simulink subsystem "MPC3_nlpsol_ipopt"  (R2023b)
settings: Solver=VariableStepAuto  StartTime=0.0  StopTime=10.0  RelTol=1e-3
undefined symbols (not defined in the file): param_MPC3_ipopt_nlpsol, param_weight_MPC3_ipopt_nlpsol, parMHE
settings Model: Creator=emu  LastModifiedBy=emu

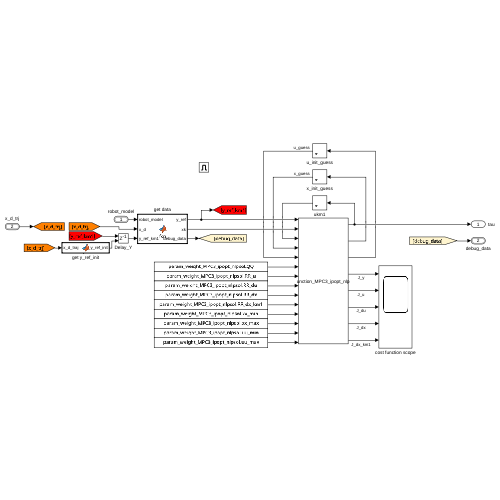
[thumbnail: Simulink's stored preview of the top-level diagram]
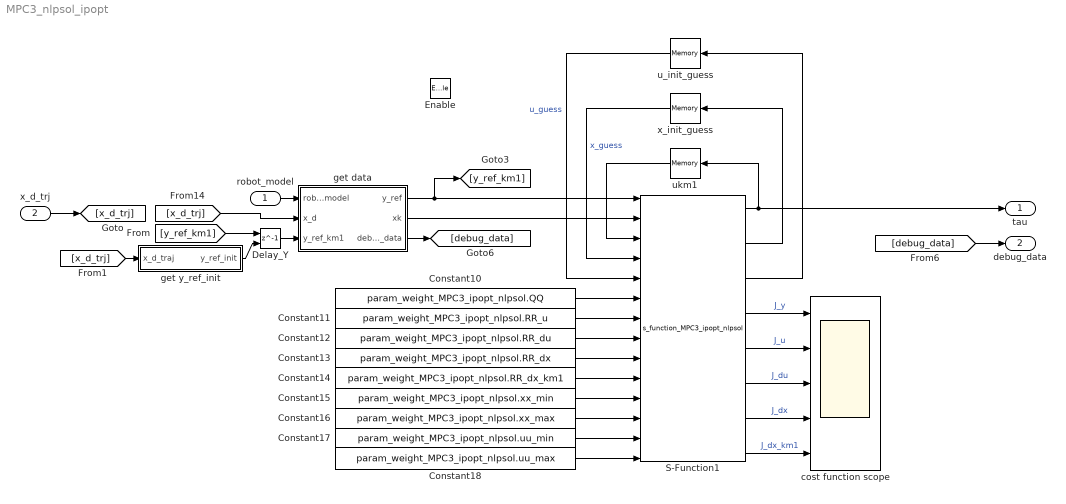
== system MPC3_nlpsol_ipopt ==
  robot_model : Inport  OutDataTypeStr=Bus: robot_model
  x_d_trj : Inport  Port=2  OutDataTypeStr=Bus: x_d
  Enable : EnablePort
  Constant10 : Constant  Value=param_weight_MPC3_ipopt_nlpsol.QQ
  Constant11 : Constant  Value=param_weight_MPC3_ipopt_nlpsol.RR_u
  Constant12 : Constant  Value=param_weight_MPC3_ipopt_nlpsol.RR_du
  Constant13 : Constant  Value=param_weight_MPC3_ipopt_nlpsol.RR_dx
  Constant14 : Constant  Value=param_weight_MPC3_ipopt_nlpsol.RR_dx_km1
  Constant15 : Constant  Value=param_weight_MPC3_ipopt_nlpsol.xx_min
  Constant16 : Constant  Value=param_weight_MPC3_ipopt_nlpsol.xx_max
  Constant17 : Constant  Value=param_weight_MPC3_ipopt_nlpsol.uu_min
  Constant18 : Constant  Value=param_weight_MPC3_ipopt_nlpsol.uu_max
  Delay_Y : Delay  DelayLength=1  InitialConditionSource=Input port  InitialCondition=zeros(parMHE.N*parMHE.n_y,1)
      settings: InputPortMap=u0,p4
  S-Function1 : S-Function  FunctionName=s_function_MPC3_ipopt_nlpsol  Parameters='s_functions/MPC3_ipopt_nlpsol.casadi', 'MPC3_ipopt_nlpsol'  SFunctionDeploymentMode=off  EnableBusSupport=off
  cost function scope : Scope  NumInputPorts=5
  get data : MATLAB Function  TreatAsAtomicUnit=on
  get y_ref_init : MATLAB Function  TreatAsAtomicUnit=on
  u_init_guess : Memory  InitialCondition=param_MPC3_ipopt_nlpsol.u_init_guess
  ukm1 : Memory  InitialCondition=param_MPC3_ipopt_nlpsol.u_init_guess(:,1)
  x_init_guess : Memory  InitialCondition=param_MPC3_ipopt_nlpsol.x_init_guess
  tau : Outport
  debug_data : Outport  Port=2  OutDataTypeStr=Bus: debug_data_bus
  wires:
  Constant15/1 -> S-Function1/11
  [y_ref_km1] -> Delay_Y/1
  u_init_guess/1 -> S-Function1/5  "u_guess"
  [x_d_trj] -> get y_ref_init/1(x_d_traj)
  Constant11/1 -> S-Function1/7
  S-Function1/1 -> ukm1/1, tau/1
  get data/1(y_ref) -> S-Function1/1, [y_ref_km1]
  x_d_trj/1 -> [x_d_trj]
  robot_model/1 -> get data/1(robot_model)
  get data/3(debug_data) -> [debug_data]
  [debug_data] -> debug_data/1
  S-Function1/4 -> cost function scope/1  "J_y"
  S-Function1/3 -> u_init_guess/1
  S-Function1/5 -> cost function scope/2  "J_u"
  get data/2(xk) -> S-Function1/2
  [x_d_trj] -> get data/2(x_d)
  ukm1/1 -> S-Function1/3
  x_init_guess/1 -> S-Function1/4  "x_guess"
  Constant18/1 -> S-Function1/14
  get y_ref_init/1(y_ref_init) -> Delay_Y/2
  Constant12/1 -> S-Function1/8
  Delay_Y/1 -> get data/3(y_ref_km1)
  S-Function1/2 -> x_init_guess/1
  Constant10/1 -> S-Function1/6
  S-Function1/7 -> cost function scope/4  "J_dx"
  S-Function1/8 -> cost function scope/5  "J_dx_km1"
  Constant17/1 -> S-Function1/13
  Constant14/1 -> S-Function1/10
  Constant13/1 -> S-Function1/9
  Constant16/1 -> S-Function1/12
  S-Function1/6 -> cost function scope/3  "J_du"

== matlab function MPC3_nlpsol_ipopt/get data ==
  settings: updateMethod=DISCRETE  sampleTime=param_global.Ta
  data: y_ref output; robot_model input Bus: robot_model; x_d input Bus: x_d; xk output; debug_data output Bus: debug_data_bus; y_ref_km1 input
function [y_ref, xk, debug_data] = fcn(robot_model,x_d, y_ref_km1)

% Parameters
q = robot_model.q;      % generalized coordinates
q_p = robot_model.q_p;  % time derivative of generalized coordinates
H = robot_model.H;

% Current Pose of Endeffector
p = H(1:3,4);
R = H(1:3,1:3);

% desired Orientation as Rotationmatrix
q_e = rotation2quaternion(R);

% Error of Position (translation) and first time derivative
q_err = quat_mult(q_e, quat_inv(x_d.q_d));

xk = [q;q_p];

% Assemble vector of recieved output measurements
Y_collected = [y_ref_km1(:,2:end) x_d.p_d(1:2)]; % 2:N+1 von trajektorie
y_ref = Y_collected;

%% DEBUG
debug_data.x = p(1);
debug_data.x_d = y_ref_km1(1,1); % aktueller wert
debug_data.y =  p(2);
debug_data.y_d = y_ref_km1(2,1); % aktueller wert
debug_data.z =  p(3);
debug_data.z_d = x_d.p_d(3);
debug_data.rot_x_err = q_err(2);
debug_data.rot_y_err = q_err(3);
debug_data.rot_z_err = q_err(4);

== matlab function MPC3_nlpsol_ipopt/get y_ref_init ==
  data: x_d_traj input; y_ref_init output; param_MPC3_ipopt_nlpsol parameter
function y_ref_init = fcn(x_d_traj, param_MPC3_ipopt_nlpsol)

y_ref_init = x_d_traj.p_d(1:2) * ones(1, param_MPC3_ipopt_nlpsol.N);
